simulink model "pi_speed_control"  (R2021b)
settings: Solver=VariableStepAuto  StartTime=0.0  StopTime=10.0  RelTol=1e-3
values from neighbouring files (symbols this model uses):
  cpr = 4096    [untitled.m]
undefined symbols (not defined in the file or in its folder): BlockInfo, ParamInfo, PortInfo, TimeInfo
libraries: simulink x1
settings Model: Creator=JongBeom  LastModifiedBy=JongBeom

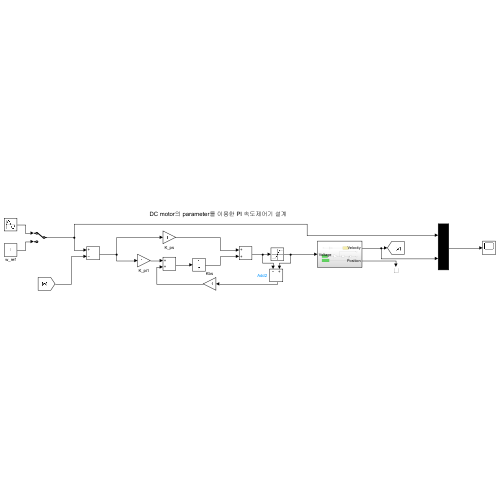
[thumbnail: Simulink's stored preview of the top-level diagram]
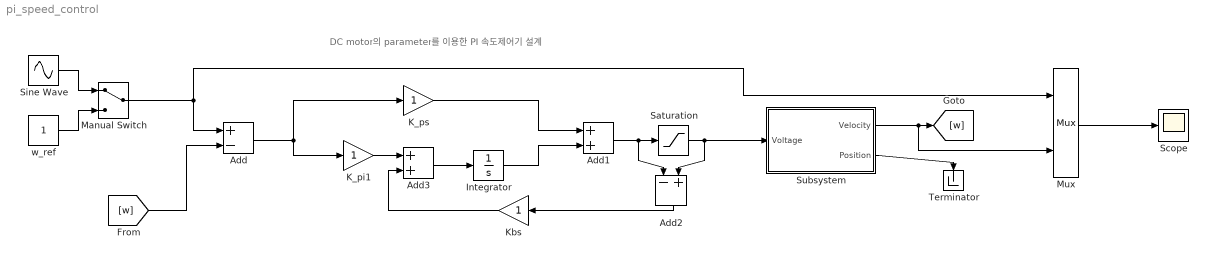
== system pi_speed_control ==
  note: DC motor의 parameter를 이용한 PI 속도제어기 설계
  Add : Sum  Inputs=+-
  Add1 : Sum
  Add2 : Sum  Inputs=-+
  Add3 : Sum
  Integrator : Integrator
  K_pi1 : Gain
  K_ps : Gain
  Kbs : Gain
  Manual Switch : ManualSwitch
  Mux : Mux  Inputs=2
  Saturation : Saturate  UpperLimit=12  LowerLimit=-12
  Scope : Scope
  Sine Wave : Sin  SampleTime=0
  Subsystem : Subsystem
  Terminator : Terminator
  w_ref : Constant
  wires:
  K_ps/1 -> Add1/1
  Integrator/1 -> Add1/2
  Add1/1 -> Add2/1, Saturation/1
  Saturation/1 -> Subsystem/1(Voltage), Add2/2
  Add2/1 -> Kbs/1
  Subsystem/1(Velocity) -> Mux/2, [w]
  [w] -> Add/2
  K_pi1/1 -> Add3/1
  Add3/1 -> Integrator/1
  Kbs/1 -> Add3/2
  Add/1 -> K_ps/1, K_pi1/1
  Subsystem/2(Position) -> Terminator/1
  Mux/1 -> Scope/1
  Sine Wave/1 -> Manual Switch/1
  w_ref/1 -> Manual Switch/2
  Manual Switch/1 -> Add/1, Mux/1

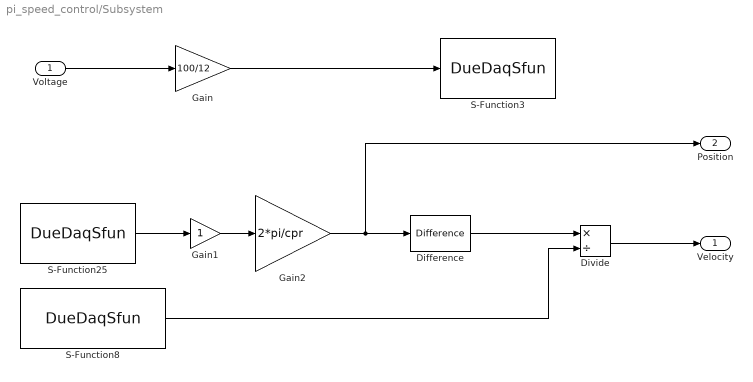
== system pi_speed_control/Subsystem ==
  Voltage : Inport
  Difference : simulink/Discrete/Difference  ICPrevInput=0.0  OutMin=[]  OutMax=[]  OutDataType=fixdt(1, 16)  OutScaling=2^-10  DoSatur=off
  Divide : Product  Inputs=*/
  Gain : Gain  Gain=100/12
  Gain1 : Gain
  Gain2 : Gain  Gain=2*pi/cpr
  S-Function25 : S-Function  FunctionName=DueDaqSfun  Parameters=TimeInfo,BlockInfo,ParamInfo,PortInfo  SFunctionDeploymentMode=off  EnableBusSupport=off  mask(Encoder Block){channel=0}
      mask prompts: channel "Channel Number"
      mask help: Receive encoder count value from Arduino Due
      mask init:
      | DueDaqRcp_Encoder_callback;
      mask TypeOptions channel: 0 | 1
      mask Display:
      | color('black');text(0.05,0.5,'(Due RCP)','horizontalalignment','left');
      | color('black');port_label('output', 1,  ' ENC0');
  S-Function3 : S-Function  FunctionName=DueDaqSfun  Parameters=TimeInfo,BlockInfo,ParamInfo,PortInfo  SFunctionDeploymentMode=off  EnableBusSupport=off  mask(PWM Block){channel=0, method=PWM/Direction, sync=off, freq=20, dead_time=3}
      mask prompts: channel "Channel Number"; sync "Synchronization with Channel 0"; freq "Frequency (KHz)"; dead_time "Dead Time"
      mask help: Send PWM information to Arduino Due
      mask init:
      | DueDaqRcp_PWM_callback;
      mask TypeOptions channel: 0 | 1 | 2 | 3 | 4 | 5
      mask Callback channel: DueDaqRcp_PWM_callback;
      mask TypeOptions method: PWM/Direction | Complementary PWM
      mask Callback method: DueDaqRcp_PWM_callback;
      mask TypeOptions freq: 1 | 10 | 20
      mask Display:
      | color('black');text(0.95,0.5,'(Due RCP)','horizontalalignment','right');
      | color('black');port_label('input', 1,  ' PWM0')
  S-Function8 : S-Function  FunctionName=DueDaqSfun  Parameters=TimeInfo,BlockInfo,ParamInfo,PortInfo  SFunctionDeploymentMode=off  EnableBusSupport=off  mask(Time Data Block){time_data_type=Time Difference}
      mask prompts: time_data_type "Time Data Type"
      mask help: Receive time-related data from Arduino Due
      mask init:
      | DueDaqRcp_TimeDiff_callback;
      mask TypeOptions time_data_type: Time | Time Difference
      mask Display:
      | color('black');text(0.05,0.5,'(Due RCP)','horizontalalignment','left');
      | color('black');port_label('output', 1,  ' TIME DIFF   ')
  Velocity : Outport
  Position : Outport  Port=2
  wires:
  Voltage/1 -> Gain/1
  Gain/1 -> S-Function3/1
  Difference/1 -> Divide/1
  Divide/1 -> Velocity/1
  S-Function25/1 -> Gain1/1
  S-Function8/1 -> Divide/2
  Gain1/1 -> Gain2/1
  Gain2/1 -> Position/1, Difference/1
